simulink model "combustion"  (R2018a)
settings: Solver=VariableStepAuto  StartTime=0.0  StopTime=10.0  RelTol=1e-3
settings Model: Creator=Lenovo  LastModifiedBy=Lenovo

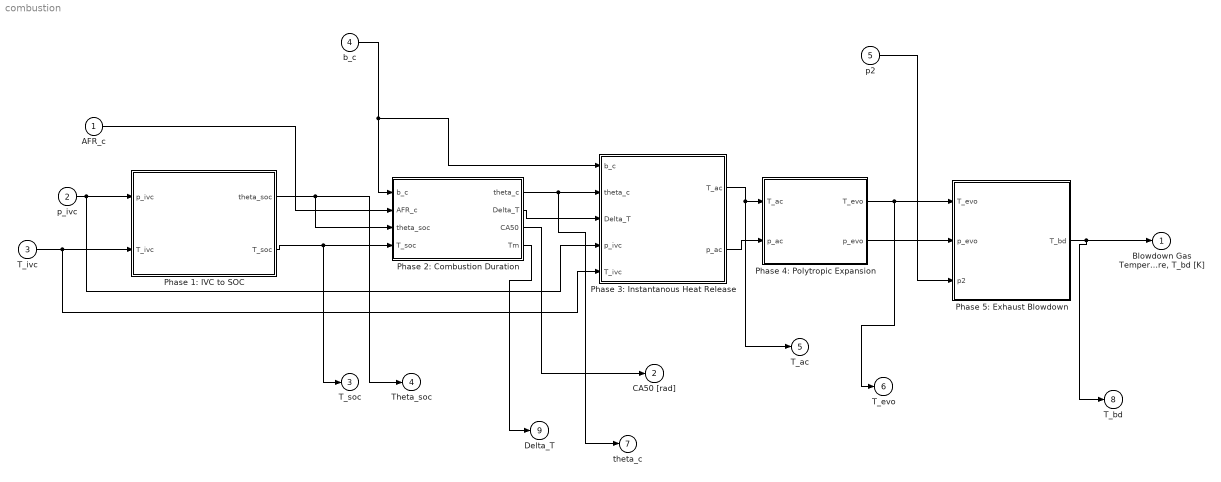
== system combustion ==
  AFR_c : Inport
  p_ivc : Inport  Port=2
  T_ivc : Inport  Port=3
  b_c : Inport  Port=4
  p2 : Inport  Port=5
  Phase 1: IVC to SOC : MATLAB Function  TreatAsAtomicUnit=on
  Phase 2: Combustion Duration : MATLAB Function  TreatAsAtomicUnit=on
  Phase 3: Instantanous Heat Release : MATLAB Function  TreatAsAtomicUnit=on
  Phase 4: Polytropic Expansion : MATLAB Function  TreatAsAtomicUnit=on
  Phase 5: Exhaust Blowdown : MATLAB Function  TreatAsAtomicUnit=on
  "Blowdown Gas Temperature, T_bd [K]" : Outport
  CA50 [rad] : Outport  Port=2
  T_soc : Outport  Port=3
  Theta_soc : Outport  Port=4
  T_ac : Outport  Port=5
  T_evo : Outport  Port=6
  theta_c : Outport  Port=7
  T_bd : Outport  Port=8
  Delta_T : Outport  Port=9
  wires:
  Phase 3: Instantanous Heat Release/1(T_ac) -> T_ac/1, Phase 4: Polytropic Expansion/1(T_ac)
  Phase 5: Exhaust Blowdown/1(T_bd) -> T_bd/1, "Blowdown Gas Temperature, T_bd [K]"/1
  Phase 2: Combustion Duration/3(CA50) -> CA50 [rad]/1
  Phase 3: Instantanous Heat Release/2(p_ac) -> Phase 4: Polytropic Expansion/2(p_ac)
  Phase 2: Combustion Duration/1(theta_c) -> theta_c/1, Phase 3: Instantanous Heat Release/2(theta_c)
  Phase 2: Combustion Duration/2(Delta_T) -> Phase 3: Instantanous Heat Release/3(Delta_T)
  AFR_c/1 -> Phase 2: Combustion Duration/2(AFR_c)
  Phase 4: Polytropic Expansion/1(T_evo) -> T_evo/1, Phase 5: Exhaust Blowdown/1(T_evo)
  Phase 1: IVC to SOC/1(theta_soc) -> Theta_soc/1, Phase 2: Combustion Duration/3(theta_soc)
  T_ivc/1 -> Phase 1: IVC to SOC/2(T_ivc), Phase 3: Instantanous Heat Release/5(T_ivc)
  Phase 4: Polytropic Expansion/2(p_evo) -> Phase 5: Exhaust Blowdown/2(p_evo)
  Phase 1: IVC to SOC/2(T_soc) -> T_soc/1, Phase 2: Combustion Duration/4(T_soc)
  p_ivc/1 -> Phase 1: IVC to SOC/1(p_ivc), Phase 3: Instantanous Heat Release/4(p_ivc)
  b_c/1 -> Phase 3: Instantanous Heat Release/1(b_c), Phase 2: Combustion Duration/1(b_c)
  p2/1 -> Phase 5: Exhaust Blowdown/3(p2)
  Phase 2: Combustion Duration/4(Tm) -> Delta_T/1

== matlab function combustion/Phase 2: Combustion Duration ==
  data: b_c input; AFR_c input; theta_soc input; theta_c output; Delta_T output; T_soc input; CA50 output; Tm output
function [theta_c, Delta_T, CA50, Tm] = duration(b_c, AFR_c, theta_soc, T_soc)
%% Arrhenius Intergral Params
A           = 3570e-5; % Arrhenius scaling constant
n           = 1.35; % reaction’s sensitivity to pressure REF2[10]
Ea          = 6317; % Arrhenius activation energy
R           = 296.25; % gas constant, J/KgK
%% Combustion Duration Params
bk0         = 0.162; % const term in k parametrization 
bk1         = 0.005; % Linear term in k dependence on theta_soc 
bk2         = 0.001; % Square term in k dependence on theta_soc

a0          = 1.0327; % Constant term in e parametrization 
a1          = -5.45; % Linear term, e dependence on k 

cv          = 1.4; % constant volume specific heat (KJ/Kg.K) [17]
Q_LHV       = 43960; % low heating value of the fuel (KJ/Kg)

Ec          = 185; % Activation energy, kJ/mol
Ru          = 8.314; % Universal gas constant, J/mol K
nc          = 1.30; % Polytropic constant during compression
ne          = 1.35; % Polytropic constant during expansion

dT_bd       = -65; % Blowdown temperature difference  
%% Params for cylinder
V_d         = 5.5e-4; % Stroke (displacement) Volume, m^3
CR          = 14; % Cylinder compression ratio
V_TDC        = V_d / (CR - 1); % Vc when piston at TDC, m^3
%% Params for cylinder (Calculated)
B           = 8.6e-2; % Bore Diameter, m
r           = 2*V_d/(pi*B^2); % Crankshaft radius, m
rod_ratio   = 1.54; % GM L61 Ecotec Engine (2.2L);
l           = rod_ratio*2*r; % Connecting rod length
%% Solve theta_soc
syms theta T;
s           = r*(1-cos(theta)+l/r*(1-sqrt(1-(r*sin(theta)/l)^2))); % stroke, m
Vc          = V_TDC + s*pi*B^2/4;

theta_ivc   = -140*pi/180; % Crank angle at IVC, rad (Fig. 5)
theta_evo   = 130*pi/180; % Crank angle at EVO, rad (Fig. 5)
V_ivc       = double(subs(Vc, theta, theta_ivc));% Cylinder Volume of Intake Valve Closing (DBC), m^3
%% Calculation
k           = bk0 + bk1*theta_soc + bk2*theta_soc^2;
e           = a0 + a1*k;
Delta_T     = Q_LHV/cv/(1+AFR_c);
Tm          = T_soc + e*(1-b_c)*Delta_T;% effective mean temperature
Delta_theta = k*T_soc^(-2/3)*Tm^(1/3)*exp(Ec/(3*Ru*Tm));

theta_c     = theta_soc + Delta_theta;
CA50        = theta_soc + 0.55*Delta_theta;

== matlab function combustion/Phase 1: IVC to SOC ==
  data: theta_soc output; p_ivc input; T_ivc input; T_soc output
function [theta_soc, T_soc]= AR_solver(p_ivc, T_ivc)
% p_ivc in Pa, T_ivc in K
%% Arrhenius Intergral Params
A           = 3570e-5; % Arrhenius scaling constant
n           = 1.35; % reaction’s sensitivity to pressure REF2[10]
Ea          = 6317; % Arrhenius activation energy
R           = 296.25; % gas constant, J/KgK
%% Combustion Duration Params
bk0         = 0.162; % const term in k parametrization 
bk1         = 0.005; % Linear term in k dependence on theta_soc 
bk2         = 0.001; % Square term in k dependence on theta_soc

a0          = 1.0327; % Constant term in e parametrization 
a1          = -5.45; % Linear term, e dependence on k 

cv          = 1.4; % constant volume specific heat (KJ/Kg.K) [17]
Q_LHV       = 43960; % low heating value of the fuel (KJ/Kg)

Ec          = 185; % Activation energy, kJ/mol
Ru          = 8.314; % Universal gas constant, J/mol K
nc          = 1.30; % Polytropic constant during compression
ne          = 1.35; % Polytropic constant during expansion

dT_bd       = -65; % Blowdown temperature difference  
%% Params for cylinder
V_d         = 5.5e-4; % Stroke (displacement) Volume, m^3
CR          = 14; % Cylinder compression ratio
V_TDC        = V_d / (CR - 1); % Vc when piston at TDC, m^3
%% Params for cylinder (Calculated)
B           = 8.6e-2; % Bore Diameter, m
r           = 2*V_d/(pi*B^2); % Crankshaft radius, m
rod_ratio   = 1.54; % GM L61 Ecotec Engine (2.2L);
l           = rod_ratio*2*r; % Connecting rod length
%% Solve theta_soc
syms theta T;
s           = r*(1-cos(theta)+l/r*(1-sqrt(1-(r*sin(theta)/l)^2))); % stroke, m
Vc          = V_TDC + s*pi*B^2/4;

theta_ivc   = -140*pi/180; % Crank angle at IVC, rad (Fig. 5)
theta_evo   = 130*pi/180; % Crank angle at EVO, rad (Fig. 5)
V_ivc       = double(subs(Vc, theta, theta_ivc));% Cylinder Volume of Intake Valve Closing (DBC), m^3
%% Calculate theta SOC
RR_theta    = A*(p_ivc^n)*(V_ivc/Vc)^(nc*n)*exp(-(Ea*(V_ivc/Vc)^(1-nc))/(R*T_ivc));

threshold   = 0.01;
step_len    = 0.001;
T           = theta_ivc:step_len:20*pi/180;
Riemann_sum = 0;

for i = 1:size(T,2)
    % v = double(subs(V_ivc/Vc, theta, T(i)))
    Riemann_sum = Riemann_sum + step_len * double(subs(RR_theta, theta, T(i)));
    disp(Riemann_sum);
    if abs(Riemann_sum - 1) <= threshold
        theta_soc = T(i);
        break
    end
end

v_soc       = double(subs(V_ivc/Vc, theta, theta_soc));
T_soc       = T_ivc*v_soc^(nc-1);
%p_soc       = R*T_soc*mc/(V_ivc/v_soc);

== matlab function combustion/Phase 3: Instantanous Heat Release ==
  data: T_ac output; p_ac output; b_c input; theta_c input; Delta_T input; p_ivc input; T_ivc input
function [T_ac, p_ac] = heat_release(b_c, theta_c, Delta_T, p_ivc, T_ivc)
%% Params for Arrhenius Integral & Combustion
%% Arrhenius Intergral Params
A           = 3570e-5; % Arrhenius scaling constant
n           = 1.35; % reaction’s sensitivity to pressure REF2[10]
Ea          = 6317; % Arrhenius activation energy
R           = 296.25; % gas constant, J/KgK
%% Combustion Duration Params
bk0         = 0.162; % const term in k parametrization 
bk1         = 0.005; % Linear term in k dependence on theta_soc 
bk2         = 0.001; % Square term in k dependence on theta_soc

a0          = 1.0327; % Constant term in e parametrization 
a1          = -5.45; % Linear term, e dependence on k 

cv          = 1.4; % constant volume specific heat (KJ/Kg.K) [17]
Q_LHV       = 43960; % low heating value of the fuel (KJ/Kg)

Ec          = 185; % Activation energy, kJ/mol
Ru          = 8.314; % Universal gas constant, J/mol K
nc          = 1.30; % Polytropic constant during compression
ne          = 1.35; % Polytropic constant during expansion

dT_bd       = -65; % Blowdown temperature difference  
%% Params for cylinder
V_d         = 5.5e-4; % Stroke (displacement) Volume, m^3
CR          = 14; % Cylinder compression ratio
V_TDC        = V_d / (CR - 1); % Vc when piston at TDC, m^3
%% Params for cylinder (Calculated)
B           = 8.6e-2; % Bore Diameter, m
r           = 2*V_d/(pi*B^2); % Crankshaft radius, m
rod_ratio   = 1.54; % GM L61 Ecotec Engine (2.2L);
l           = rod_ratio*2*r; % Connecting rod length
%% Solve theta_soc
syms theta T;
s           = r*(1-cos(theta)+l/r*(1-sqrt(1-(r*sin(theta)/l)^2))); % stroke, m
Vc          = V_TDC + s*pi*B^2/4;

theta_ivc   = -140*pi/180; % Crank angle at IVC, rad (Fig. 5)
theta_evo   = 130*pi/180; % Crank angle at EVO, rad (Fig. 5)
V_ivc       = double(subs(Vc, theta, theta_ivc));% Cylinder Volume of Intake Valve Closing (DBC), m^3
%% Params Before Combustion 
T_bc        = T_ivc*double(subs(V_ivc/Vc, theta, theta_c))^(nc-1);
p_bc        = p_ivc*double(subs(V_ivc/Vc, theta, theta_c))^nc;
%% Params After Combustion
T_ac        = T_bc + (1-b_c)*Delta_T;
p_ac        = p_bc*T_ac/T_bc;

== matlab function combustion/Phase 4: Polytropic Expansion ==
  data: T_evo output; p_evo output; T_ac input; p_ac input
function [T_evo, p_evo] = expansion(T_ac, p_ac)
%% Params for Arrhenius Integral & Combustion
%% Arrhenius Intergral Params
A           = 3570e-5; % Arrhenius scaling constant
n           = 1.35; % reaction’s sensitivity to pressure REF2[10]
Ea          = 6317; % Arrhenius activation energy
R           = 296.25; % gas constant, J/KgK
%% Combustion Duration Params
bk0         = 0.162; % const term in k parametrization 
bk1         = 0.005; % Linear term in k dependence on theta_soc 
bk2         = 0.001; % Square term in k dependence on theta_soc

a0          = 1.0327; % Constant term in e parametrization 
a1          = -5.45; % Linear term, e dependence on k 

cv          = 1.4; % constant volume specific heat (KJ/Kg.K) [17]
Q_LHV       = 43960; % low heating value of the fuel (KJ/Kg)

Ec          = 185; % Activation energy, kJ/mol
Ru          = 8.314; % Universal gas constant, J/mol K
nc          = 1.30; % Polytropic constant during compression
ne          = 1.35; % Polytropic constant during expansion

dT_bd       = -65; % Blowdown temperature difference  
%% Params for cylinder
V_d         = 5.5e-4; % Stroke (displacement) Volume, m^3
CR          = 14; % Cylinder compression ratio
V_TDC        = V_d / (CR - 1); % Vc when piston at TDC, m^3
%% Params for cylinder (Calculated)
B           = 8.6e-2; % Bore Diameter, m
r           = 2*V_d/(pi*B^2); % Crankshaft radius, m
rod_ratio   = 1.54; % GM L61 Ecotec Engine (2.2L);
l           = rod_ratio*2*r; % Connecting rod length
%% Solve theta_soc
syms theta T;
s           = r*(1-cos(theta)+l/r*(1-sqrt(1-(r*sin(theta)/l)^2))); % stroke, m
Vc          = V_TDC + s*pi*B^2/4;

theta_ivc   = -140*pi/180; % Crank angle at IVC, rad (Fig. 5)
theta_evo   = 130*pi/180; % Crank angle at EVO, rad (Fig. 5)
V_ivc       = double(subs(Vc, theta, theta_ivc));% Cylinder Volume of Intake Valve Closing (DBC), m^3
%% Calculation
T_evo        = T_ac*double(subs(V_ivc/Vc, theta, theta_evo))^(ne-1);
p_evo        = p_ac*double(subs(V_ivc/Vc, theta, theta_evo))^ne;

== matlab function combustion/Phase 5: Exhaust Blowdown ==
  data: T_bd output; T_evo input; p_evo input; p2 input
function T_bd = blowdowm(T_evo, p_evo, p2)
%% Params for Arrhenius Integral & Combustion
%% Arrhenius Intergral Params
A           = 3570e-5; % Arrhenius scaling constant
n           = 1.35; % reaction’s sensitivity to pressure REF2[10]
Ea          = 6317; % Arrhenius activation energy
R           = 296.25; % gas constant, J/KgK
%% Combustion Duration Params
bk0         = 0.162; % const term in k parametrization 
bk1         = 0.005; % Linear term in k dependence on theta_soc 
bk2         = 0.001; % Square term in k dependence on theta_soc

a0          = 1.0327; % Constant term in e parametrization 
a1          = -5.45; % Linear term, e dependence on k 

cv          = 1.4; % constant volume specific heat (KJ/Kg.K) [17]
Q_LHV       = 43960; % low heating value of the fuel (KJ/Kg)

Ec          = 185; % Activation energy, kJ/mol
Ru          = 8.314; % Universal gas constant, J/mol K
nc          = 1.30; % Polytropic constant during compression
ne          = 1.35; % Polytropic constant during expansion

dT_bd       = -65; % Blowdown temperature difference  
%% Params for cylinder
V_d         = 5.5e-4; % Stroke (displacement) Volume, m^3
CR          = 14; % Cylinder compression ratio
V_TDC        = V_d / (CR - 1); % Vc when piston at TDC, m^3
%% Params for cylinder (Calculated)
B           = 8.6e-2; % Bore Diameter, m
r           = 2*V_d/(pi*B^2); % Crankshaft radius, m
rod_ratio   = 1.54; % GM L61 Ecotec Engine (2.2L);
l           = rod_ratio*2*r; % Connecting rod length
%% Solve theta_soc
syms theta T;
s           = r*(1-cos(theta)+l/r*(1-sqrt(1-(r*sin(theta)/l)^2))); % stroke, m
Vc          = V_TDC + s*pi*B^2/4;

theta_ivc   = -140*pi/180; % Crank angle at IVC, rad (Fig. 5)
theta_evo   = 130*pi/180; % Crank angle at EVO, rad (Fig. 5)
V_ivc       = double(subs(Vc, theta, theta_ivc));% Cylinder Volume of Intake Valve Closing (DBC), m^3
%% Params Before Combustion 
T_bd        = T_evo*(p2/p_evo)^((ne-1)/ne) + dT_bd;
